simulink model "simplified_magnet19"  (R2019b)
settings: Solver=FixedStepDiscrete  StartTime=0.0  StopTime=5  FixedStep=Ts  RelTol=1e-3
InitFcn:
  | init_simulink
values from neighbouring files (symbols this model uses):
  Ad = dplantsys.a    [init_simulink.m]
  Bd = dplantsys.b    [init_simulink.m]
  Cd = dplantsys.c    [init_simulink.m]
  Dd = dplantsys.d    [init_simulink.m]
  Kfb = dlqr(Alqr, Blqr, Q, R)    [init_simulink.m]
  Ts = 1.25e-2    (= 0.0125)    [init_simulink.m]
undefined symbols (not defined in the file or in its folder): DiscIntNeverNeededParam
libraries: simulink x1
settings Model: Creator=ayeiser  LastModifiedBy=josh
settings OptimizationCC: PassReuseOutputArgsAs=Individual arguments  OptimizeBlockOrder=speed  DifferentSizesBufferReuse=on  EfficientTunableParamExpr=on
settings DebuggingCC: ParameterTunabilityLossMsg=error
settings HardwareCC: TargetBitPerLong=64  TargetBitPerPointer=64  TargetBitPerSizeT=64  TargetBitPerPtrDiffT=64  TargetLongLongMode=on  TargetIntDivRoundTo=Zero  TargetEndianess=LittleEndian  TargetWordSize=64  TargetHWDeviceType=MATLAB Host  ProdEqTarget=off
settings SFSimCC: MATLABDynamicMemAlloc=off
settings RTWCC: Description=Embedded Coder (host-based shared library target)  SystemTargetFile=ert_shrlib.tlc  TemplateMakefile=ert_default_tmf  RTWVerbose=off  CustomDefine=-DTHIS_MODEL_NAME=$(PRODUCT_NAME)
settings RTWCC: CustomSourceCode=|
  | #define CONCAT(str1, str2, str3) CONCAT_(str1, str2, str3)
  | #define CONCAT_(str1, str2, str3) str1 ## str2 ## str3
  | #define GET_MMI_FUNC    CONCAT(THIS_MODEL_NAME, _GetCAPImmi    ,   )
  | #define RT_MODEL_STRUCT CONCAT(RT_MODEL_      , THIS_MODEL_NAME, _T)
  | 
  | void* GET_MMI_FUNC(void* voidPtrToRealTimeStructure)
  | {
  |    rtwCAPI_ModelMappingInfo* mmiPtr = &(rtmGetDataMapInfo( ( RT_MODEL_STRUCT * )(voidPtrToRealTimeStructure) ).mmi);
  |    return (void*) mmiPtr;
  | }
settings CodeAppCC: ForceParamTrailComments=on  GenerateComments=off  IgnoreCustomStorageClasses=off  OperatorAnnotations=on  SimulinkDataObjDesc=on  SFDataObjDesc=on  InsertBlockDesc=on
settings STFCustomTargetCC: TargetLangStandard=C99 (ISO)  MultiwordLength=256  ParMdlRefBuildCompliant=on  CompOptLevelCompliant=on  IncludeMdlTerminateFcn=off  CombineOutputUpdateFcns=on  CombineSignalStateStructs=on  SuppressErrorStatus=on  ERTCustomFileBanners=on  SupportAbsoluteTime=off  MultiInstanceERTCode=on  CodeInterfacePackaging=Reusable function  SupportComplex=off  SupportContinuousTime=off  SupportNonInlinedSFcns=off  RemoveResetFunc=on  MATLABClassNameForMDSCustomization=Simulink.SoftwareTarget.ERTCustomization  ModelStepFunctionPrototypeControlCompliant=on  GenerateAllocFcn=on  UseToolchainInfoCompliant=on  SystemTargetFile=ert_shrlib.tlc
settings ERTTargetCC: TargetLangStandard=C99 (ISO)  ConcurrentExecutionCompliant=off  IncludeMdlTerminateFcn=off  CombineSignalStateStructs=on  SuppressErrorStatus=on  SupportAbsoluteTime=off  MultiInstanceERTCode=on  CodeInterfacePackaging=Reusable function  SupportComplex=off  CPPClassGenCompliant=off  GenerateAllocFcn=on  RootIOFormat=Part of model data structure  RTWCAPIParams=on  RTWCAPIRootIO=on  ERTCustomFileTemplate=example_file_process.tlc

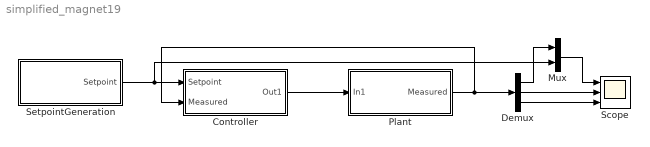
== system simplified_magnet19 ==
  Controller : Subsystem
  Demux : Demux  Outputs=3
  Mux : Mux  Inputs=2
  Plant : Subsystem
  Scope : Scope  NumInputPorts=3
  SetpointGeneration : Subsystem
  wires:
  SetpointGeneration/1(Setpoint) -> Mux/2, Controller/1(Setpoint)
  Plant/1(Measured) -> Demux/1, Controller/2(Measured)
  Demux/2 -> Scope/2
  Demux/3 -> Scope/3
  Mux/1 -> Scope/1
  Demux/1 -> Mux/1
  Controller/1(Out1) -> Plant/1(In1)

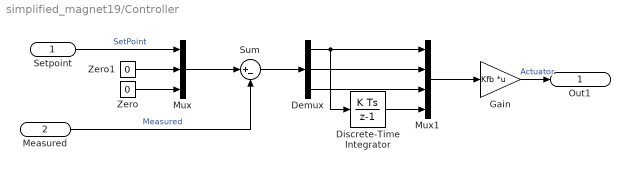
== system simplified_magnet19/Controller ==
  Setpoint : Inport
  Measured : Inport  Port=2  PortDimensions=3
  Demux : Demux  Outputs=3
  Discrete-Time Integrator : DiscreteIntegrator  SampleTime=-1  ICPrevOutput=DiscIntNeverNeededParam  ICPrevScaledInput=DiscIntNeverNeededParam
  Gain : Gain  Gain=Kfb  Multiplication=Matrix(K*u)
  Mux : Mux  Inputs=3
  Mux1 : Mux
  Sum : Sum  Inputs=|+-
  Zero : Constant  Value=0  OutDataTypeStr=Inherit: Inherit via back propagation
  Zero1 : Constant  Value=0  OutDataTypeStr=Inherit: Inherit via back propagation
  Out1 : Outport  PortDimensions=1
  wires:
  Zero/1 -> Mux/3
  Zero1/1 -> Mux/2
  Mux/1 -> Sum/1
  Measured/1 -> Sum/2  "Measured"
  Gain/1 -> Out1/1  "Actuator"
  Sum/1 -> Demux/1
  Demux/1 -> Mux1/1, Discrete-Time Integrator/1
  Demux/2 -> Mux1/2
  Demux/3 -> Mux1/3
  Discrete-Time Integrator/1 -> Mux1/4
  Mux1/1 -> Gain/1
  Setpoint/1 -> Mux/1  "SetPoint"

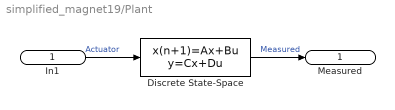
== system simplified_magnet19/Plant ==
  In1 : Inport  PortDimensions=1
  Discrete State-Space : DiscreteStateSpace  A=Ad  B=Bd  C=Cd  D=Dd  SampleTime=Ts
  Measured : Outport  PortDimensions=3
  wires:
  In1/1 -> Discrete State-Space/1  "Actuator"
  Discrete State-Space/1 -> Measured/1  "Measured"

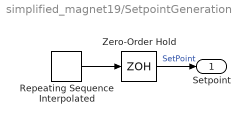
== system simplified_magnet19/SetpointGeneration ==
  Repeating Sequence Interpolated : simulink/Sources/Repeating Sequence Interpolated  OutValues=[0 0 0.01 0.01].'  TimeValues=[0 1 1.01 5].'  LookUpMeth=Interpolation-Use End Values  tsamp=Ts  OutMin=[]  OutMax=[]  OutDataTypeStr=double  OutputDataTypeScalingMode=double  OutDataType=fixdt(0,8)  OutScaling=2^-10
  Zero-Order Hold : ZeroOrderHold  SampleTime=-1
  Setpoint : Outport
  wires:
  Repeating Sequence Interpolated/1 -> Zero-Order Hold/1
  Zero-Order Hold/1 -> Setpoint/1  "SetPoint"
